simulink model "simulation"  (R2022b)
settings: Solver=VariableStepAuto  StartTime=0.0  StopTime=7200  RelTol=1e-3
undefined symbols (not defined in the file): sigbuilder_block
libraries: slpidlib x1, dspstat3 x1
settings Model: Creator=Anvitha  LastModifiedBy=Anvitha

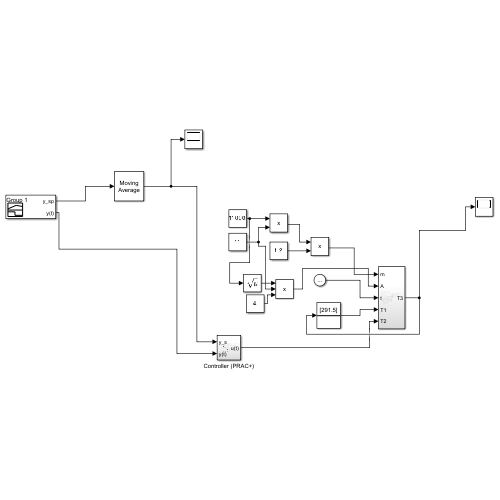
[thumbnail: Simulink's stored preview of the top-level diagram]
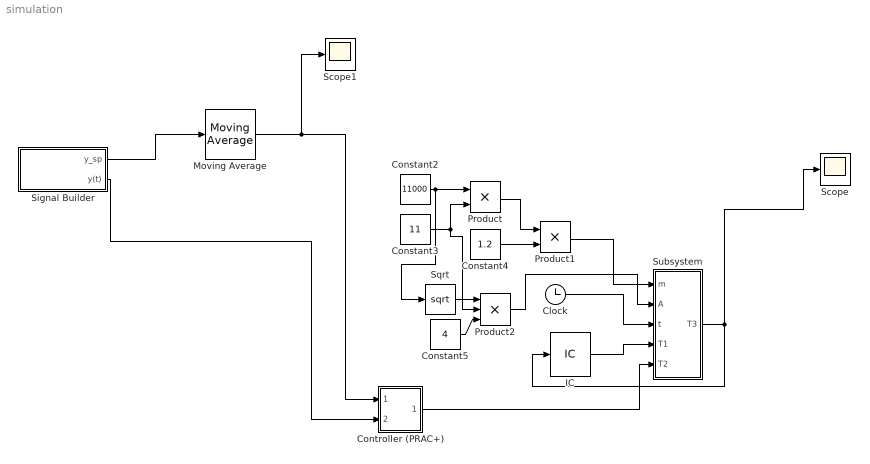
== system simulation ==
  Clock : Clock
      settings: Decimation=1000
  Constant2 : Constant  Value=11000
  Constant3 : Constant  Value=11
  Constant4 : Constant  Value=1.2
  Constant5 : Constant  Value=4
  Controller (PRAC+) : Subsystem
  IC : InitialCondition  Value=291.5
  Moving Average : dspstat3/Moving Average  Method=Exponential weighting  ForgettingFactorPort=off  SpecifyWindowLength=on  WindowLength=4  OverlapLength=3  AllowArbitraryInputLength=off  ForgettingFactor=0.99  SimulateUsing=Code generation
  Product : Product
  Product1 : Product
  Product2 : Product  Inputs=3
  Scope : Scope
  Scope1 : Scope
  Signal Builder : Subsystem  Tag=STV Subsys  LoadFcn=sigbuilder_block('load');  StartFcn=sigbuilder_block('start');  StopFcn=sigbuilder_block('stop');  ClipboardFcn=sigbuilder_block('clipboard');  mask(Sigbuilder block){tuvar=[0:10]}
      mask help: Simulink:masks:SigbuilderBlock_MD
      mask init:
      | if ~strcmp(get_param(bdroot(gcbh),'SimulationStatus'),'stopped') tuvar = sigbuilder_block('maskInit'); end
      settings: CopyFcn=sigbuilder_block('copy');  DeleteFcn=sigbuilder_block('delete');  ModelCloseFcn=sigbuilder_block('modelClose');  PreSaveFcn=sigbuilder_block('preSave');  PauseFcn=sigbuilder_block('pause');  ContinueFcn=sigbuilder_block('continue');  NameChangeFcn=sigbuilder_block('namechange');  OpenFcn=sigbuilder_block('open',[-28 67.5 949 412 ]);  CloseFcn=sigbuilder_block('close');
      mask Display: plot(0, 0, 100, 100,[2, 2, 32, 32, 2], [68, 8, 8, 68, 68],[32, 2], [38, 38], [32, 19, 2],[53, 60, 44], [32, 17, 17, 2],[16, 16, 31, 31]);txt = getActiveGroup(gcbh);text(2, 100, txt,'verticalAlignment', 'top');
  Sqrt : Sqrt
  Subsystem : Subsystem
  wires:
  IC/1 -> Subsystem/4(T1)
  Constant2/1 -> Sqrt/1, Product/1
  Constant3/1 -> Product2/2, Product/2
  Constant4/1 -> Product1/2
  Product/1 -> Product1/1
  Product1/1 -> Subsystem/1(m)
  Sqrt/1 -> Product2/1
  Constant5/1 -> Product2/3
  Product2/1 -> Subsystem/2(A)
  Clock/1 -> Subsystem/3(t)
  Signal Builder/2(y(t)) -> Controller (PRAC+)/2(y(t))
  Subsystem/1(T3) -> IC/1, Scope/1
  Controller (PRAC+)/1(u(t)) -> Subsystem/5(T2)
  Signal Builder/1(y_sp) -> Moving Average/1
  Moving Average/1 -> Scope1/1, Controller (PRAC+)/1(y_s)

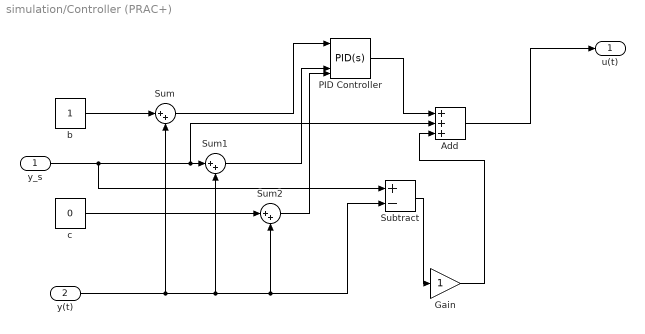
== system simulation/Controller (PRAC+) ==
  y_s : Inport
  y(t) : Inport  Port=2
  Add : Sum  Inputs=+++
  Gain : Gain
  PID Controller : slpidlib/PID Controller  Controller=PID  Form=Ideal  TimeDomain=Continuous-time  UseExternalTs=off  SampleTime=-1  IntegratorMethod=Forward Euler  FilterMethod=Forward Euler  ControllerParametersSource=external  P=1  I=1  UseKiTs=off  D=0  N=100  UseFilter=on  TunerSelectOption=Transfer Function Based (PID Tuner App)  InitialConditionSource=external  InitialConditionForIntegrator=0  InitialConditionForFilter=0  DifferentiatorICPrevScaledInput=0  ExternalReset=none  TrackingMode=off  Kt=1  LimitOutput=on  SatLimitsSource=internal  UpperSaturationLimit=20  LowerSaturationLimit=0  LinearizeAsGain=off  AntiWindupMode=back-calculation  Kb=1  LimitIntegrator=off  UpperIntegratorSaturationLimit=inf  LowerIntegratorSaturationLimit=-inf  RndMeth=Nearest  POutMin=[]  POutMax=[]  IOutMin=[]  IOutMax=[]  DOutMin=[]  DOutMax=[]  NOutMin=[]  NOutMax=[]  SumOutMin=[]  SumOutMax=[]  SaturationOutMin=[]  SaturationOutMax=[]  PParamMin=[]  PParamMax=[]  IParamMin=[]  IParamMax=[]  DParamMin=[]  DParamMax=[]  NParamMin=[]  NParamMax=[]  KbParamMin=[]  KbParamMax=[]  KtParamMin=[]  KtParamMax=[]  KbOutMin=[]  KbOutMax=[]  KtOutMin=[]  KtOutMax=[]  IntegratorOutMin=[]  IntegratorOutMax=[]  FilterOutMin=[]  FilterOutMax=[]  SumI1OutMin=[]  SumI1OutMax=[]  SumI2OutMin=[]  SumI2OutMax=[]  SumI3OutMin=[]  SumI3OutMax=[]  SumI4OutMin=[]  SumI4OutMax=[]  SumDOutMin=[]  SumDOutMax=[]  DifferentiatorOutMin=[]  DifferentiatorOutMax=[]  FilterDiffOutCoefMin=[]  FilterDiffOutCoefMax=[]  ReciprocalOutMin=[]  ReciprocalOutMax=[]  SumDenOutMin=[]  SumDenOutMax=[]  SumNumOutMin=[]  SumNumOutMax=[]  DivideOutMin=[]  DivideOutMax=[]  UdiffTsProdOutMin=[]  UdiffTsProdOutMax=[]  NTsProdOutMin=[]  NTsProdOutMax=[]  UintegralTsProdOutMin=[]  UintegralTsProdOutMax=[]  UngainTsProdOutMin=[]  UngainTsProdOutMax=[]  ClampingZeroOutDataTypeStr=Inherit: Inherit via back propagation  ClampingZeroOutMin=[]  ClampingZeroOutMax=[]  FilterDenConstantOutDataTypeStr=Inherit: Inherit via back propagation  FilterDenConstantOutMin=[]  FilterDenConstantOutMax=[]  PCopyOutDataTypeStr=Inherit: Inherit via back propagation  PCopyOutMin=[]  PCopyOutMax=[]  NCopyOutDataTypeStr=Inherit: Inherit via back propagation  NCopyOutMin=[]  NCopyOutMax=[]  IntegratorContinuousStateAttributes=''  IntegratorStateMustResolveToSignalObject=off  IntegratorRTWStateStorageClass=Auto  FilterContinuousStateAttributes=''  FilterStateMustResolveToSignalObject=off  FilterRTWStateStorageClass=Auto  ParallelPVariant=Passthrough  IdealPVariant=ExternalParameters  IVariant=ExternalParameters  DVariant=ExternalParameters  IntegratorVariant=Continuous  SatVariant=Enabled  AWVariant=BackCalculation  PCopyVariant=Disabled  TRVariant=Disabled  FdbkBlocksVariant=Forward  IdealPFdbkVariant=Disabled  SatFdbkVariant=Disabled  DerivativeFilterVariant=ContFilter  NVariant=ExternalParameters  NCopyVariant=Disabled  FilterICVariant=ExternalICs  IntegratorICVariant=ExternalICs  ExternalResetVariant=Disabled  TRSumVariant=Passthrough  SumFdbkVariant=Disabled  SumVariant=Sum_PID  TsampFilterVariant=InternalTs  TsampNgainVariant=Passthrough  TsampIntegralVariant=Passthrough  ExternalSaturationOutDataTypeStr=Inherit: Same as second input
  Subtract : Sum  Inputs=+-
  Sum : Sum  Inputs=|++
  Sum1 : Sum  Inputs=|++
  Sum2 : Sum  Inputs=|++
  b : Constant
  c : Constant  Value=0
  u(t) : Outport
  wires:
  y_s/1 -> Subtract/1, Add/2, Sum1/1
  Sum2/1 -> PID Controller/7
  b/1 -> Sum/1
  y(t)/1 -> Subtract/2, Sum2/2, Sum1/2, Sum/2
  Sum/1 -> PID Controller/1
  Sum1/1 -> PID Controller/6
  c/1 -> Sum2/1
  PID Controller/1 -> Add/1
  Add/1 -> u(t)/1
  Subtract/1 -> Gain/1
  Gain/1 -> Add/3

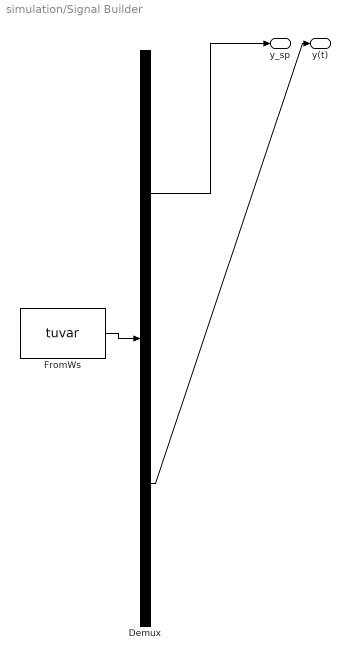
== system simulation/Signal Builder ==
  Demux : Demux  Tag=STV Demux  Outputs=2
      settings: DisplayOption=none
  FromWs : FromWorkspace  Tag=STV FromWs  VariableName=tuvar
      SigBuilderData=|
      | common.afterFinalStr = 'Extrapolate'
      | common.sampleTime = 0
      | dataSet.timeRange = [0 7200]
      | dataSet.name = 'Group 1'
      | sbobj.Groups.Name = 'Group 1'
      | sbobj.Groups.Signals(1).Name = 'y_sp'
      | sbobj.Groups.Signals(1).XData = [0 800 800 1600 1600 2400 2400 3200 3200 4000 4000 4800 4800 5600 5600 6400 6400 7200]
      | sbobj.Groups.Signals(1).YData = [295 295 291.5 291.5 295 295 291.5 291.5 295 295 291.5 291.5 295 295 291.5 291.5 295 295]
      | sbobj.Groups.Signals(2).Name = 'y(t)'
      | sbobj.Groups.Signals(2).XData = [0 7200]
      | sbobj.Groups.Signals(2).YData = [291.5 291.5]
      | sbobj.Groups.TimeRange = [0 7200]
  y_sp : Outport  Tag=STV Outport
  y(t) : Outport  Tag=STV Outport  Port=2
  wires:
  FromWs/1 -> Demux/1
  Demux/1 -> y_sp/1
  Demux/2 -> y(t)/1

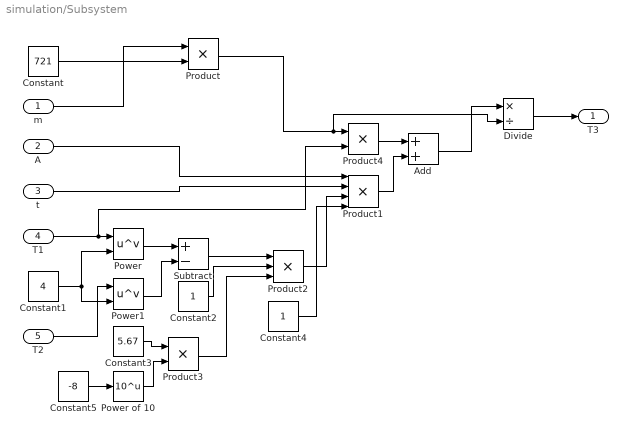
== system simulation/Subsystem ==
  m : Inport
  A : Inport  Port=2
  t : Inport  Port=3
  T1 : Inport  Port=4
  T2 : Inport  Port=5
  Add : Sum  Inputs=2
  Constant : Constant  Value=721
  Constant1 : Constant  Value=4
  Constant2 : Constant
  Constant3 : Constant  Value=5.67
  Constant4 : Constant
  Constant5 : Constant  Value=-8
  Divide : Product  Inputs=*/
  Power : Math  Operator=pow
  Power of 10 : Math  Operator=10^u
  Power1 : Math  Operator=pow
  Product : Product
  Product1 : Product  Inputs=4
  Product2 : Product  Inputs=3
  Product3 : Product
  Product4 : Product
  Subtract : Sum  Inputs=+-
  T3 : Outport
  wires:
  Product4/1 -> Add/1
  Constant2/1 -> Product2/2
  Constant3/1 -> Product3/1
  Power1/1 -> Subtract/2
  T1/1 -> Product4/2, Power/1
  Constant1/1 -> Power1/2, Power/2
  Constant5/1 -> Power of 10/1
  m/1 -> Product/1
  Product2/1 -> Product1/3
  Add/1 -> Divide/1
  t/1 -> Product1/2
  Subtract/1 -> Product2/1
  T2/1 -> Power1/1
  Product/1 -> Divide/2, Product4/1
  Product1/1 -> Add/2
  Product3/1 -> Product2/3
  Constant/1 -> Product/2
  Power/1 -> Subtract/1
  Divide/1 -> T3/1
  A/1 -> Product1/1
  Power of 10/1 -> Product3/2
  Constant4/1 -> Product1/4
